simulink model "read_current_and_motor_driver"  (R2021b)
settings: Solver=ode1  StartTime=0.0  StopTime=120  FixedStep=0.01  RelTol=1e-3  EnableMultiTasking=on
libraries: arduinolib x6, arduinosensorlib x1
settings Model: ExtModeTrigDuration=2  Creator=ASUS  LastModifiedBy=ASUS
settings OptimizationCC: EnhancedBackFolding=on  PassReuseOutputArgsAs=Individual arguments  ZeroExternalMemoryAtStartup=off  ZeroInternalMemoryAtStartup=off  MaxStackSize=64  OptimizeBlockOrder=speed  DifferentSizesBufferReuse=on  OptimizationCustomize=off  EfficientTunableParamExpr=on
settings DebuggingCC: ParameterTunabilityLossMsg=error
settings HardwareCC: ProdBitPerInt=16  ProdBitPerPointer=16  ProdBitPerSizeT=16  ProdBitPerPtrDiffT=16  ProdLargestAtomicFloat=None  ProdWordSize=8  ProdHWDeviceType=Atmel->AVR
settings SFSimCC: MATLABDynamicMemAlloc=off
settings RTWCC: Description=Embedded Coder  SystemTargetFile=ert.tlc  HardwareBoard=Arduino Mega 2560  TemplateMakefile=ert_default_tmf  Toolchain=Arduino AVR  BuildConfiguration=Faster Runs
settings CodeAppCC: ForceParamTrailComments=on  IgnoreCustomStorageClasses=off  OperatorAnnotations=on  SimulinkDataObjDesc=on  SFDataObjDesc=on  InsertBlockDesc=on
settings ERTTargetCC: SupportContinuousTime=on  SupportVariableSizeSignals=on  ExtModeTransport=3  ExtModeStaticAlloc=on  ExtModeStaticAllocSize=2048  ExtModeMexFile=ext_xcp  ExtModeIntrfLevel=Level2 - Open

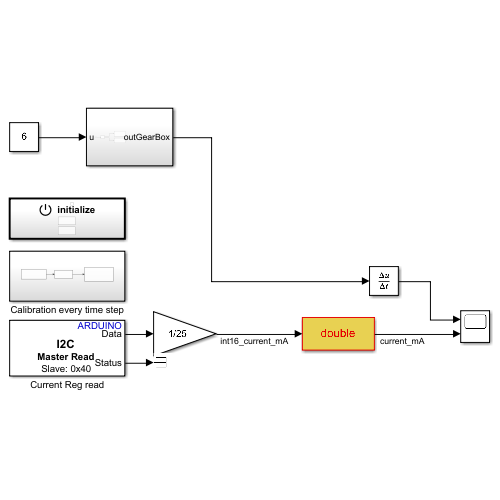
[thumbnail: Simulink's stored preview of the top-level diagram]
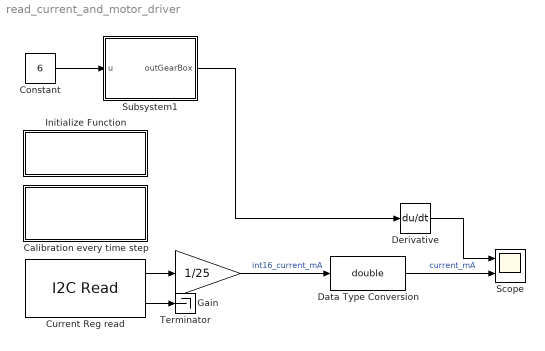
== system read_current_and_motor_driver ==
  Calibration every time step : Subsystem  Priority=0
  Constant : Constant  Value=6
  Current Reg read : arduinolib/I2C Read  I2CModule=0  Mode=Master  SlaveAddress="hex2dec(\"0x40\")"  SlaveByteOrder=BigEndian  Direction=Receiver  RegisterAddressMode=on  RegisterAddress="hex2dec(\"0x04\")"  SlaveDataType=int16  DataLength=1  NoAck=off  RepeatedStart=off  OutputStatus=on  blockPlatform=ARDUINO  SampleTime=0.01
      settings: SourceProductBaseCode=ARDUINO
  Data Type Conversion : DataTypeConversion  OutDataTypeStr=double
  Derivative : Derivative
  Gain : Gain  Gain=1/25
  Initialize Function : Subsystem  TreatAsAtomicUnit=on
  Scope : Scope  NumInputPorts=2
  Subsystem1 : Subsystem
  Terminator : Terminator
  wires:
  Constant/1 -> Subsystem1/1(u)
  Subsystem1/1(outGearBox) -> Derivative/1
  Derivative/1 -> Scope/1
  Gain/1 -> Data Type Conversion/1  "int16_current_mA"
  Current Reg read/1 -> Gain/1
  Current Reg read/2 -> Terminator/1
  Data Type Conversion/1 -> Scope/2  "current_mA"

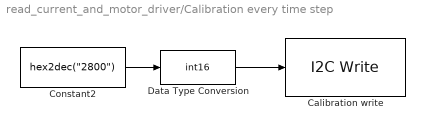
== system read_current_and_motor_driver/Calibration every time step ==
  Calibration write : arduinolib/I2C Write  I2CModule=0  Mode=Master  SlaveAddress="uint8(hex2dec(\"0x40\"))"  SlaveByteOrder=BigEndian  Direction=Transmitter  RegisterAddressMode=on  RegisterAddress="uint8(hex2dec(\"0x05\"))"  SlaveDataType=uint8  DataLength=1  NoAck=off  RepeatedStart=off  OutputStatus=off  blockPlatform=ARDUINO
      settings: SourceProductBaseCode=ARDUINO
  Constant2 : Constant  Value="hex2dec(\"2800\")"
  Data Type Conversion : DataTypeConversion  OutDataTypeStr=int16
  wires:
  Constant2/1 -> Data Type Conversion/1
  Data Type Conversion/1 -> Calibration write/1

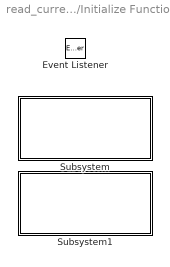
== system read_current_and_motor_driver/Initialize Function ==
  Event Listener : EventListener  DisableCoverage=on  EventName=reset
  Subsystem : Subsystem  Priority=0
  Subsystem1 : Subsystem  Priority=1

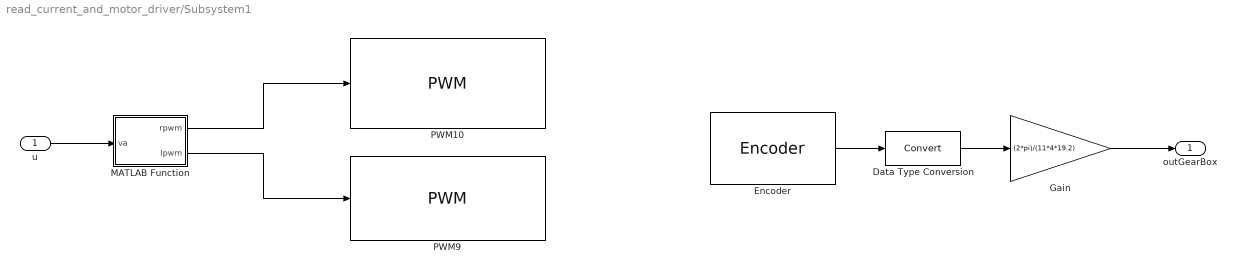
== system read_current_and_motor_driver/Subsystem1 ==
  u : Inport
  Data Type Conversion : DataTypeConversion
  Encoder : arduinosensorlib/Encoder  InputA=2  InputB=3  Mode=No reset  SampleTime=-1
      settings: SourceProductBaseCode=ARDUINO
  Gain : Gain  Gain=(2*pi)/(11*4*19.2)
  MATLAB Function : MATLAB Function  TreatAsAtomicUnit=on
  PWM10 : arduinolib/PWM  pinNumber=8  frequencyType=Default  desiredFrequency=490.2  achievableFrequency=490.2
  PWM9 : arduinolib/PWM  pinNumber=9  frequencyType=Default  desiredFrequency=490.2  achievableFrequency=490.2
  outGearBox : Outport
  wires:
  MATLAB Function/2(lpwm) -> PWM9/1
  MATLAB Function/1(rpwm) -> PWM10/1
  u/1 -> MATLAB Function/1(va)
  Encoder/1 -> Data Type Conversion/1
  Gain/1 -> outGearBox/1
  Data Type Conversion/1 -> Gain/1

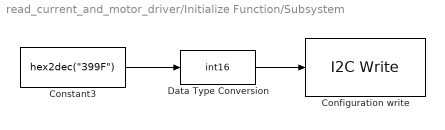
== system read_current_and_motor_driver/Initialize Function/Subsystem ==
  Configuration write : arduinolib/I2C Write  I2CModule=0  Mode=Master  SlaveAddress="hex2dec(\"0x40\")"  SlaveByteOrder=BigEndian  Direction=Transmitter  RegisterAddressMode=on  RegisterAddress="hex2dec(\"0x00\")"  SlaveDataType=uint8  DataLength=1  NoAck=off  RepeatedStart=off  OutputStatus=off  blockPlatform=ARDUINO
      settings: SourceProductBaseCode=ARDUINO
  Constant3 : Constant  Value="hex2dec(\"399F\")"
  Data Type Conversion : DataTypeConversion  OutDataTypeStr=int16
  wires:
  Constant3/1 -> Data Type Conversion/1
  Data Type Conversion/1 -> Configuration write/1

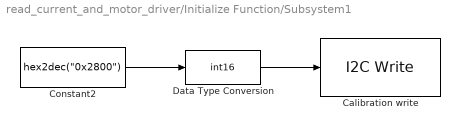
== system read_current_and_motor_driver/Initialize Function/Subsystem1 ==
  Calibration write : arduinolib/I2C Write  I2CModule=0  Mode=Master  SlaveAddress="uint8(hex2dec(\"0x40\"))"  SlaveByteOrder=BigEndian  Direction=Transmitter  RegisterAddressMode=on  RegisterAddress="uint8(hex2dec(\"0x05\"))"  SlaveDataType=uint8  DataLength=1  NoAck=off  RepeatedStart=off  OutputStatus=off  blockPlatform=ARDUINO
      settings: SourceProductBaseCode=ARDUINO
  Constant2 : Constant  Value="hex2dec(\"0x2800\")"
  Data Type Conversion : DataTypeConversion  OutDataTypeStr=int16
  wires:
  Constant2/1 -> Data Type Conversion/1
  Data Type Conversion/1 -> Calibration write/1

== matlab function read_current_and_motor_driver/Subsystem1/MATLAB Function ==
  data: va input; rpwm output; lpwm output
function [rpwm,lpwm] = fcn(va)

pwm = (va/24)*254;

if pwm > 0
    rpwm = pwm;
    lpwm = 0;
elseif pwm<0
    rpwm = 0;
    lpwm = abs(pwm);
else
    rpwm = 0;
    lpwm = 0;
end
